simulink model "log_map_sl"  (Simulink 6.4)
settings: Solver=FixedStepDiscrete  StartTime=0.0  StopTime=50.0  FixedStep=0.1  RelTol=1e-3
undefined symbols (not defined in the file or in its folder): alpha, beta, lambda, y1_0, y2_0
settings Model: LastModifiedBy=alexh  OSC_ATGCV_WORKDIR=C:\test_ground\target_link_stuff\sixth\new_profile
settings DataIOCC: LimitDataPoints=off  SaveOutput=off  SaveTime=off
settings OptimizationCC: BooleanDataType=off
settings DebuggingCC: SolverPrmCheckMsg=none  StrictBusMsg=None
settings HardwareCC: TargetUnknown=on

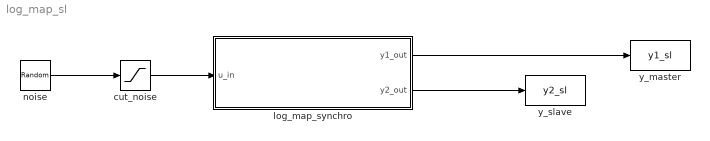
== system log_map_sl ==
  cut_noise : Saturate  UpperLimit=1  LowerLimit=0
  log_map_synchro : Subsystem
  noise : RandomNumber  Mean=0.5  SampleTime=0
  y_master : ToWorkspace  VariableName=y1_sl  SampleTime=-1  SaveFormat=Array
  y_slave : ToWorkspace  VariableName=y2_sl  SampleTime=-1  SaveFormat=Array
  wires:
  noise/1 -> cut_noise/1
  log_map_synchro/1(y1_out) -> y_master/1
  cut_noise/1 -> log_map_synchro/1(u_in)
  log_map_synchro/2(y2_out) -> y_slave/1

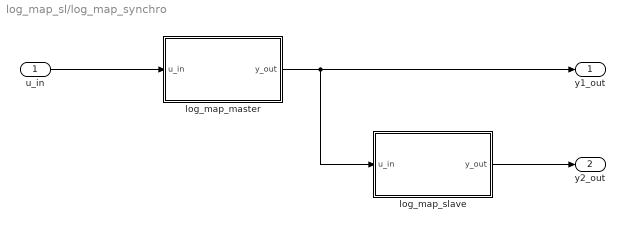
== system log_map_sl/log_map_synchro ==
  u_in : Inport
  log_map_master : Subsystem
  log_map_slave : Subsystem
  y1_out : Outport
  y2_out : Outport  Port=2
  wires:
  u_in/1 -> log_map_master/1(u_in)
  log_map_master/1(y_out) -> y1_out/1, log_map_slave/1(u_in)
  log_map_slave/1(y_out) -> y2_out/1

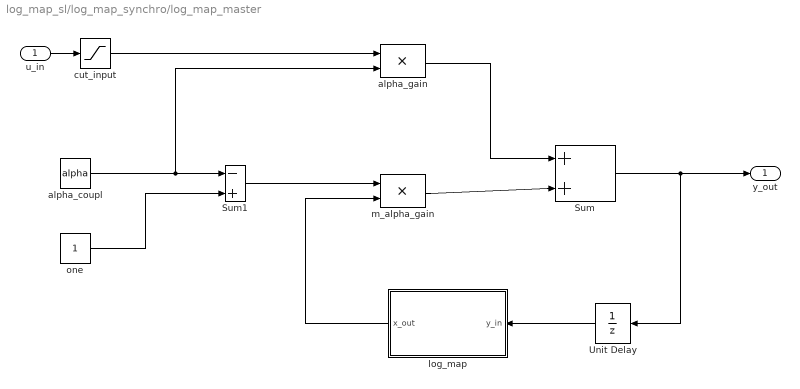
== system log_map_sl/log_map_synchro/log_map_master ==
  u_in : Inport
  Sum : Sum  Inputs=+|+  SaturateOnIntegerOverflow=on  InputSameDT=on
  Sum1 : Sum  Inputs=-|+  SaturateOnIntegerOverflow=on  InputSameDT=on
  Unit Delay : UnitDelay  Orientation=left  X0=y1_0  SampleTime=-1
  alpha_coupl : Constant  Value=alpha  OutDataType=sfix(16)  ConRadixGroup=Use specified scaling  OutScaling=2^0  SampleTime=inf  FramePeriod=inf
  alpha_gain : Product  SaturateOnIntegerOverflow=on  RndMeth=Zero  InputSameDT=on
  cut_input : Saturate  UpperLimit=1  LowerLimit=0
  log_map : Subsystem  Orientation=left
  m_alpha_gain : Product  SaturateOnIntegerOverflow=on  RndMeth=Zero  InputSameDT=on
  one : Constant  Value=1  OutDataType=sfix(16)  ConRadixGroup=Use specified scaling  OutScaling=2^0  SampleTime=inf  FramePeriod=inf
  y_out : Outport
  wires:
  alpha_gain/1 -> Sum/1
  log_map/1(x_out) -> m_alpha_gain/2
  Sum/1 -> Unit Delay/1, y_out/1
  u_in/1 -> cut_input/1
  cut_input/1 -> alpha_gain/1
  Unit Delay/1 -> log_map/1(y_in)
  m_alpha_gain/1 -> Sum/2
  one/1 -> Sum1/2
  alpha_coupl/1 -> Sum1/1, alpha_gain/2
  Sum1/1 -> m_alpha_gain/1

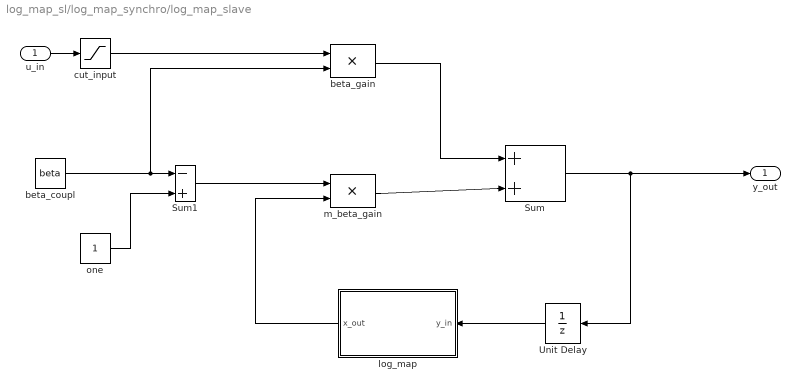
== system log_map_sl/log_map_synchro/log_map_slave ==
  u_in : Inport
  Sum : Sum  Inputs=+|+  SaturateOnIntegerOverflow=on  InputSameDT=on
  Sum1 : Sum  Inputs=-|+  SaturateOnIntegerOverflow=on  InputSameDT=on
  Unit Delay : UnitDelay  Orientation=left  X0=y2_0  SampleTime=-1
  beta_coupl : Constant  Value=beta  OutDataType=sfix(16)  ConRadixGroup=Use specified scaling  OutScaling=2^0  SampleTime=inf  FramePeriod=inf
  beta_gain : Product  SaturateOnIntegerOverflow=on  RndMeth=Zero  InputSameDT=on
  cut_input : Saturate  UpperLimit=1  LowerLimit=0
  log_map : Subsystem  Orientation=left
  m_beta_gain : Product  SaturateOnIntegerOverflow=on  RndMeth=Zero  InputSameDT=on
  one : Constant  Value=1  OutDataType=sfix(16)  ConRadixGroup=Use specified scaling  OutScaling=2^0  SampleTime=inf  FramePeriod=inf
  y_out : Outport
  wires:
  m_beta_gain/1 -> Sum/2
  Unit Delay/1 -> log_map/1(y_in)
  cut_input/1 -> beta_gain/1
  u_in/1 -> cut_input/1
  Sum/1 -> y_out/1, Unit Delay/1
  log_map/1(x_out) -> m_beta_gain/2
  beta_gain/1 -> Sum/1
  Sum1/1 -> m_beta_gain/1
  beta_coupl/1 -> Sum1/1, beta_gain/2
  one/1 -> Sum1/2

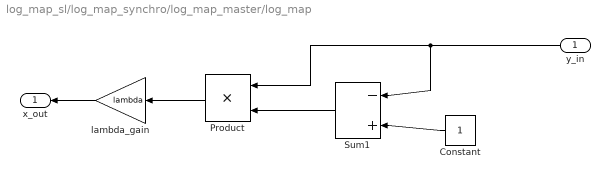
== system log_map_sl/log_map_synchro/log_map_master/log_map ==
  y_in : Inport  Orientation=left
  Constant : Constant  Orientation=left  Value=1  OutDataType=sfix(16)  ConRadixGroup=Use specified scaling  OutScaling=2^0  SampleTime=inf  FramePeriod=inf
  Product : Product  Orientation=left  SaturateOnIntegerOverflow=on  RndMeth=Zero  InputSameDT=on
  Sum1 : Sum  Orientation=left  Inputs=-|+  SaturateOnIntegerOverflow=on  InputSameDT=on
  lambda_gain : Gain  Orientation=left  Gain=lambda  SaturateOnIntegerOverflow=on
  x_out : Outport  Orientation=left
  wires:
  Constant/1 -> Sum1/2
  Sum1/1 -> Product/2
  y_in/1 -> Product/1, Sum1/1
  Product/1 -> lambda_gain/1
  lambda_gain/1 -> x_out/1

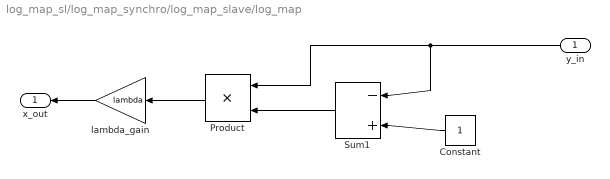
== system log_map_sl/log_map_synchro/log_map_slave/log_map ==
  y_in : Inport  Orientation=left
  Constant : Constant  Orientation=left  Value=1  OutDataType=sfix(16)  ConRadixGroup=Use specified scaling  OutScaling=2^0  SampleTime=inf  FramePeriod=inf
  Product : Product  Orientation=left  SaturateOnIntegerOverflow=on  RndMeth=Zero  InputSameDT=on
  Sum1 : Sum  Orientation=left  Inputs=-|+  SaturateOnIntegerOverflow=on  InputSameDT=on
  lambda_gain : Gain  Orientation=left  Gain=lambda  SaturateOnIntegerOverflow=on
  x_out : Outport  Orientation=left
  wires:
  lambda_gain/1 -> x_out/1
  Product/1 -> lambda_gain/1
  y_in/1 -> Sum1/1, Product/1
  Sum1/1 -> Product/2
  Constant/1 -> Sum1/2
